simulink model "SS_elastico_SP19"  (R2024b)
settings: Solver=VariableStepAuto  StartTime=0.0  StopTime=tsamplesimulink  RelTol=1e-3
undefined symbols (not defined in the file): Ac, Bcg, Cc, Dcg, g, Je, Jm, Ka, Kfd, Kfp, Km, Kp, Kv, m, N, tm, xc
settings Model: Creator=Isaac  LastModifiedBy=ruizh
settings SolverCC: AlgebraicLoopSolver=TrustRegion
settings DataIOCC: ReturnWorkspaceOutputs=off
settings DebuggingCC: UnconnectedInputMsg=warning  UnconnectedOutputMsg=warning  UnconnectedLineMsg=warning  ArithmeticOperatorsInVariantConditions=warning
settings ModelReferenceCC: EnableRefExpFcnMdlSchedulingChecks=on
settings SFSimCC: SimUseLocalCustomCode=off  CustomCodeUndefinedFunction=UseInterfaceOnly
settings RTWCC: RTWUseLocalCustomCode=off  GPUComputeCapability=3.5
settings CodeAppCC: StateflowObjectComments=on

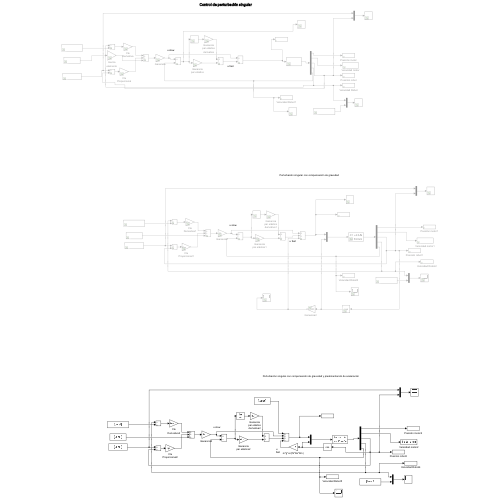
[thumbnail: Simulink's stored preview of the top-level diagram]
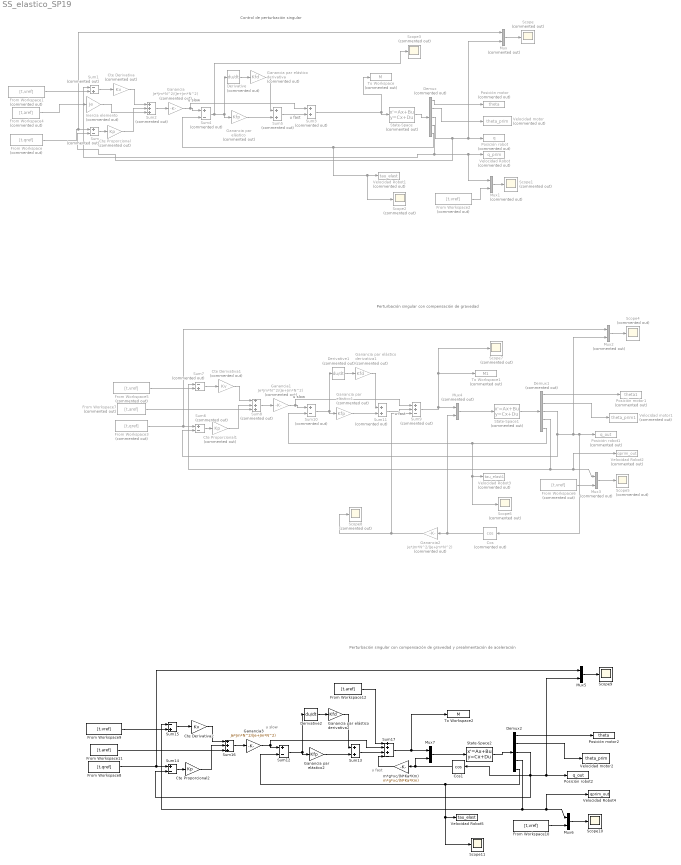
== system SS_elastico_SP19 ==
  note: Control de perturbación singular
  note: Perturbación singular con compensación de gravedad
  note: u fast
  note: u slow
  note: u fast
  note: u slow
  note: Perturbación singular con compensación de gravedad y prealimentación de aceleración
  note: u fast
  note: u slow
  Cos : Trigonometry  Commented=on  Operator=cos
  Cos1 : Trigonometry  Operator=cos
  Cte Derivativa : Gain  Commented=on  Gain=Kv  SaturateOnIntegerOverflow=on  OutDataTypeStr=Inherit: Same as input  ParamDataTypeStr=Inherit: Same as input
  Cte Derivativa1 : Gain  Commented=on  Gain=Kv  SaturateOnIntegerOverflow=on  OutDataTypeStr=Inherit: Same as input  ParamDataTypeStr=Inherit: Same as input
  Cte Derivativa2 : Gain  Gain=Kv  SaturateOnIntegerOverflow=on  OutDataTypeStr=Inherit: Same as input  ParamDataTypeStr=Inherit: Same as input
  Cte Proporcional : Gain  Commented=on  Gain=Kp  SaturateOnIntegerOverflow=on  OutDataTypeStr=Inherit: Same as input  ParamDataTypeStr=Inherit: Same as input
  Cte Proporcional1 : Gain  Commented=on  Gain=Kp  SaturateOnIntegerOverflow=on  OutDataTypeStr=Inherit: Same as input  ParamDataTypeStr=Inherit: Same as input
  Cte Proporcional2 : Gain  Gain=Kp  SaturateOnIntegerOverflow=on  OutDataTypeStr=Inherit: Same as input  ParamDataTypeStr=Inherit: Same as input
  Demux : Demux  Commented=on  Outputs=5
  Demux1 : Demux  Commented=on  Outputs=5
  Demux2 : Demux  Outputs=5
  Derivative : Derivative  Commented=on
  Derivative1 : Derivative  Commented=on
  Derivative2 : Derivative
  From Workspace : FromWorkspace  Commented=on  VariableName=[t,qref]  SampleTime=tm  ZeroCross=off
  From Workspace{1..2,5..6} (4 alike) : FromWorkspace  Commented=on  VariableName=[t,vref]  SampleTime=tm  ZeroCross=off
  From Workspace10 : FromWorkspace  VariableName=[t,vref]  SampleTime=tm  ZeroCross=off
  From Workspace11 : FromWorkspace  VariableName=[t,aref]  SampleTime=tm  ZeroCross=off
  From Workspace12 : FromWorkspace  VariableName=[t,aref]  SampleTime=tm  ZeroCross=off
  From Workspace3 : FromWorkspace  Commented=on  VariableName=[t,qref]  SampleTime=tm  ZeroCross=off
  From Workspace4 : FromWorkspace  Commented=on  VariableName=[t,aref]  SampleTime=tm  ZeroCross=off
  From Workspace7 : FromWorkspace  Commented=on  VariableName=[t,aref]  SampleTime=tm  ZeroCross=off
  From Workspace8 : FromWorkspace  VariableName=[t,qref]  SampleTime=tm  ZeroCross=off
  From Workspace9 : FromWorkspace  VariableName=[t,vref]  SampleTime=tm  ZeroCross=off
  Ganancia : Gain  Commented=on  Gain=Je*Jm*N^2/(Je+Jm*N^2)  SaturateOnIntegerOverflow=on  OutDataTypeStr=Inherit: Same as input  ParamDataTypeStr=Inherit: Same as input
  Ganancia par elástico : Gain  Commented=on  Gain=Kfp  SaturateOnIntegerOverflow=on  OutDataTypeStr=Inherit: Same as input  ParamDataTypeStr=Inherit: Same as input
  Ganancia par elástico derivativa : Gain  Commented=on  Gain=Kfd  SaturateOnIntegerOverflow=on  OutDataTypeStr=Inherit: Same as input  ParamDataTypeStr=Inherit: Same as input
  Ganancia par elástico derivativa1 : Gain  Commented=on  Gain=Kfd  SaturateOnIntegerOverflow=on  OutDataTypeStr=Inherit: Same as input  ParamDataTypeStr=Inherit: Same as input
  Ganancia par elástico derivativa2 : Gain  Gain=Kfd  SaturateOnIntegerOverflow=on  OutDataTypeStr=Inherit: Same as input  ParamDataTypeStr=Inherit: Same as input
  Ganancia par elástico1 : Gain  Commented=on  Gain=Kfp  SaturateOnIntegerOverflow=on  OutDataTypeStr=Inherit: Same as input  ParamDataTypeStr=Inherit: Same as input
  Ganancia par elástico2 : Gain  Gain=Kfp  SaturateOnIntegerOverflow=on  OutDataTypeStr=Inherit: Same as input  ParamDataTypeStr=Inherit: Same as input
  Ganancia1 : Gain  Commented=on  Gain=Je*Jm*N^2/(Je+Jm*N^2)  SaturateOnIntegerOverflow=on  OutDataTypeStr=Inherit: Same as input  ParamDataTypeStr=Inherit: Same as input
  Ganancia2 : Gain  Commented=on  Gain=Je*Jm*N^2/(Je+Jm*N^2)  SaturateOnIntegerOverflow=on  OutDataTypeStr=Inherit: Same as input  ParamDataTypeStr=Inherit: Same as input
  Ganancia3 : Gain  Gain=Je*Jm*N^2/(Je+Jm*N^2)  SaturateOnIntegerOverflow=on  OutDataTypeStr=Inherit: Same as input  ParamDataTypeStr=Inherit: Same as input
  Inercia elemento : Gain  Commented=on  Gain=Je  SaturateOnIntegerOverflow=on  OutDataTypeStr=Inherit: Same as input  ParamDataTypeStr=Inherit: Same as input
  Mux{,1..4} (5 alike) : Mux  Commented=on  Inputs=2
  Mux5 : Mux  Inputs=2
  Mux6 : Mux  Inputs=2
  Mux7 : Mux  Inputs=2
  Posición motor : ToWorkspace  Commented=on  VariableName=theta  SampleTime=tm
  Posición motor1 : ToWorkspace  Commented=on  VariableName=theta1  SampleTime=tm
  Posición motor2 : ToWorkspace  VariableName=theta  SampleTime=tm
  Posición robot : ToWorkspace  Commented=on  VariableName=q  SampleTime=tm
  Posición robot1 : ToWorkspace  Commented=on  VariableName=q_out  SampleTime=tm
  Posición robot2 : ToWorkspace  VariableName=q_out  SampleTime=tm
  Scope{,1..8} (9 alike) : Scope  Commented=on
  Scope10 : Scope
  Scope11 : Scope
  Scope9 : Scope
  State-Space : StateSpace  Commented=on  A=Ac  B=Bcg  C=Cc  D=Dcg  InitialCondition=0
  State-Space1 : StateSpace  Commented=on  A=Ac  B=Bcg  C=Cc  D=Dcg  InitialCondition=0
  State-Space2 : StateSpace  A=Ac  B=Bcg  C=Cc  D=Dcg  InitialCondition=0
  Sum{,4,6,10} (4 alike) : Sum  Commented=on  Inputs=+-  InputSameDT=on  SaturateOnIntegerOverflow=on  OutDataTypeStr=Inherit: Same as first input
  Sum1 : Sum  Commented=on  Inputs=-+  InputSameDT=on  SaturateOnIntegerOverflow=on  OutDataTypeStr=Inherit: Same as first input
  Sum11 : Sum  Commented=on  InputSameDT=on  SaturateOnIntegerOverflow=on  OutDataTypeStr=Inherit: Same as first input
  Sum12 : Sum  Inputs=+-  InputSameDT=on  SaturateOnIntegerOverflow=on  OutDataTypeStr=Inherit: Same as first input
  Sum13 : Sum  InputSameDT=on  SaturateOnIntegerOverflow=on  OutDataTypeStr=Inherit: Same as first input
  Sum14 : Sum  Inputs=+-  InputSameDT=on  SaturateOnIntegerOverflow=on  OutDataTypeStr=Inherit: Same as first input
  Sum15 : Sum  Inputs=-+  InputSameDT=on  SaturateOnIntegerOverflow=on  OutDataTypeStr=Inherit: Same as first input
  Sum16 : Sum  Inputs=+++  InputSameDT=on  SaturateOnIntegerOverflow=on  OutDataTypeStr=Inherit: Same as first input
  Sum17 : Sum  Inputs=+++-  InputSameDT=on  SaturateOnIntegerOverflow=on  OutDataTypeStr=Inherit: Same as first input
  Sum2 : Sum  Commented=on  Inputs=+++  InputSameDT=on  SaturateOnIntegerOverflow=on  OutDataTypeStr=Inherit: Same as first input
  Sum3 : Sum  Commented=on  InputSameDT=on  SaturateOnIntegerOverflow=on  OutDataTypeStr=Inherit: Same as first input
  Sum5 : Sum  Commented=on  InputSameDT=on  SaturateOnIntegerOverflow=on  OutDataTypeStr=Inherit: Same as first input
  Sum7 : Sum  Commented=on  Inputs=-+  InputSameDT=on  SaturateOnIntegerOverflow=on  OutDataTypeStr=Inherit: Same as first input
  Sum8 : Sum  Commented=on  Inputs=+++  InputSameDT=on  SaturateOnIntegerOverflow=on  OutDataTypeStr=Inherit: Same as first input
  Sum9 : Sum  Commented=on  Inputs=++-  InputSameDT=on  SaturateOnIntegerOverflow=on  OutDataTypeStr=Inherit: Same as first input
  To Workspace : ToWorkspace  Commented=on  VariableName=M  SampleTime=tm
  To Workspace1 : ToWorkspace  Commented=on  VariableName=M1  SampleTime=tm
  To Workspace2 : ToWorkspace  VariableName=M  SampleTime=tm
  Velocidad Robot : ToWorkspace  Commented=on  VariableName=q_prim  SampleTime=tm
  Velocidad Robot1 : ToWorkspace  Commented=on  VariableName=tau_elast  SampleTime=tm
  Velocidad Robot2 : ToWorkspace  Commented=on  VariableName=qprim_out  SampleTime=tm
  Velocidad Robot3 : ToWorkspace  Commented=on  VariableName=tau_elast1  SampleTime=tm
  Velocidad Robot4 : ToWorkspace  VariableName=qprim_out  SampleTime=tm
  Velocidad Robot5 : ToWorkspace  VariableName=tau_elast  SampleTime=tm
  Velocidad motor : ToWorkspace  Commented=on  VariableName=theta_prim  SampleTime=tm
  Velocidad motor1 : ToWorkspace  Commented=on  VariableName=theta_prim1  SampleTime=tm
  Velocidad motor2 : ToWorkspace  VariableName=theta_prim  SampleTime=tm
  m*g*xc/(N*Ka*Km) : Gain  Gain=m*g*xc/(N*Ka*Km)  SaturateOnIntegerOverflow=on  OutDataTypeStr=Inherit: Same as input  ParamDataTypeStr=Inherit: Same as input
  wires:
  Sum3/1 -> State-Space/1, To Workspace/1
  Demux/1 -> Posición motor/1
  Cte Derivativa/1 -> Sum2/1
  From Workspace/1 -> Sum/1, Mux/1
  Sum/1 -> Cte Proporcional/1
  Cte Proporcional/1 -> Sum2/2
  Demux/4 -> Sum1/1, Mux1/1, Velocidad Robot/1
  Sum1/1 -> Cte Derivativa/1
  From Workspace1/1 -> Sum1/2
  Demux/3 -> Sum/2, Mux/2, Posición robot/1
  Mux/1 -> Scope/1
  State-Space/1 -> Demux/1
  Demux/2 -> Velocidad motor/1
  Inercia elemento/1 -> Sum2/3
  From Workspace4/1 -> Inercia elemento/1
  Sum4/1 -> Scope3/1, Derivative/1, Ganancia par elástico/1
  Demux/5 -> Scope2/1, Velocidad Robot1/1, Sum4/2
  Mux1/1 -> Scope1/1
  From Workspace2/1 -> Mux1/2
  Derivative/1 -> Ganancia par elástico derivativa/1
  Sum2/1 -> Ganancia/1
  Ganancia/1 -> Sum3/1, Sum4/1
  Ganancia par elástico derivativa/1 -> Sum5/1
  Ganancia par elástico/1 -> Sum5/2
  Sum5/1 -> Sum3/2
  Sum7/1 -> Cte Derivativa1/1
  Ganancia par elástico1/1 -> Sum11/2
  Derivative1/1 -> Ganancia par elástico derivativa1/1
  Sum11/1 -> Sum9/2
  Demux1/3 -> Sum6/2, Mux2/2, Cos/1, Posición robot1/1
  Sum9/1 -> Scope7/1, To Workspace1/1, Mux4/1
  Demux1/2 -> Velocidad motor1/1
  From Workspace5/1 -> Sum7/2
  Demux1/4 -> Sum7/1, Velocidad Robot2/1, Mux3/1
  Ganancia1/1 -> Sum9/1, Sum10/1
  Demux1/5 -> Sum10/2, Scope6/1, Velocidad Robot3/1
  Sum10/1 -> Derivative1/1, Ganancia par elástico1/1
  Cte Proporcional1/1 -> Sum8/2
  Mux3/1 -> Scope5/1
  Mux2/1 -> Scope4/1
  From Workspace3/1 -> Sum6/1, Mux2/1
  Ganancia par elástico derivativa1/1 -> Sum11/1
  Sum6/1 -> Cte Proporcional1/1
  Demux1/1 -> Posición motor1/1
  From Workspace6/1 -> Mux3/2
  Sum8/1 -> Ganancia1/1
  Cte Derivativa1/1 -> Sum8/1
  State-Space1/1 -> Demux1/1
  From Workspace7/1 -> Sum8/3
  Ganancia2/1 -> Scope8/1, Sum9/3
  Cos/1 -> Mux4/2, Ganancia2/1
  Mux4/1 -> State-Space1/1
  Mux5/1 -> Scope9/1
  Sum12/1 -> Derivative2/1, Ganancia par elástico2/1
  From Workspace11/1 -> Sum16/3
  Demux2/5 -> Sum12/2, Scope11/1, Velocidad Robot5/1
  State-Space2/1 -> Demux2/1
  Ganancia par elástico2/1 -> Sum13/2
  Mux7/1 -> State-Space2/1
  Sum17/1 -> To Workspace2/1, Mux7/1
  Demux2/3 -> Posición robot2/1, Mux5/2, Cos1/1, Sum14/2
  Ganancia3/1 -> Sum12/1, Sum17/2
  Ganancia par elástico derivativa2/1 -> Sum13/1
  From Workspace10/1 -> Mux6/2
  From Workspace9/1 -> Sum15/2
  Cte Derivativa2/1 -> Sum16/1
  Demux2/1 -> Posición motor2/1
  From Workspace8/1 -> Sum14/1, Mux5/1
  Cte Proporcional2/1 -> Sum16/2
  Cos1/1 -> Mux7/2, m*g*xc/(N*Ka*Km)/1
  Mux6/1 -> Scope10/1
  Demux2/4 -> Sum15/1, Velocidad Robot4/1, Mux6/1
  m*g*xc/(N*Ka*Km)/1 -> Sum17/4
  Sum14/1 -> Cte Proporcional2/1
  Sum15/1 -> Cte Derivativa2/1
  Sum16/1 -> Ganancia3/1
  Derivative2/1 -> Ganancia par elástico derivativa2/1
  Demux2/2 -> Velocidad motor2/1
  Sum13/1 -> Sum17/3
  From Workspace12/1 -> Sum17/1
